simulink library "SEMACE1_OUT"  (R2021b)
settings: Solver=VariableStepAuto  StartTime=0.0  StopTime=10.0  RelTol=1e-3
settings Model: Creator=ACH  LastModifiedBy=ACH

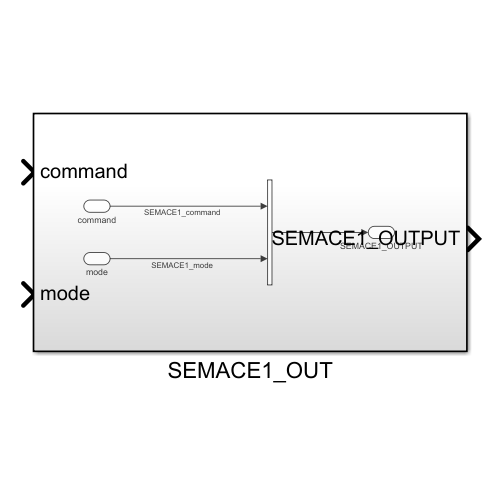
[thumbnail: Simulink's stored preview of the top-level diagram]
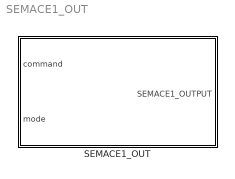
== system SEMACE1_OUT ==
  SEMACE1_OUT : Subsystem

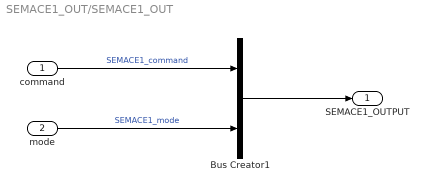
== system SEMACE1_OUT/SEMACE1_OUT ==
  command : Inport
  mode : Inport  Port=2
  Bus Creator1 : BusCreator  Inputs=2  OutDataTypeStr=Bus: SEMACE1_OUTPUT
  SEMACE1_OUTPUT : Outport  OutDataTypeStr=Bus: SEMACE1_OUTPUT
  wires:
  command/1 -> Bus Creator1/1  "SEMACE1_command"
  mode/1 -> Bus Creator1/2  "SEMACE1_mode"
  Bus Creator1/1 -> SEMACE1_OUTPUT/1
